simulink model "rSteeringAngle"  (R2024b)
settings: Solver=FixedStepAuto  StartTime=0.0  StopTime=10.0  RelTol=1e-3  EnableMultiTasking=on
undefined symbols (not defined in the file): aSteeringAngleMax, rSteeringAngleGain
settings Model: DataDictionary=Master_Dictionary.sldd  EnableAccessToBaseWorkspace=off  Creator=torni  LastModifiedBy=Will
settings OptimizationCC: DefaultParameterBehavior=Inlined  EnhancedBackFolding=on  PassReuseOutputArgsAs=Individual arguments  ZeroExternalMemoryAtStartup=off  ZeroInternalMemoryAtStartup=off  MaxStackSize=8192  OptimizeBlockOrder=speed  DifferentSizesBufferReuse=on  OptimizationCustomize=off  EfficientTunableParamExpr=on
settings DebuggingCC: ParameterTunabilityLossMsg=error
settings HardwareCC: ProdBitPerPointer=32  ProdBitPerSizeT=32  ProdBitPerPtrDiffT=32  ProdLargestAtomicInteger=Long  ProdLargestAtomicFloat=Double  ProdWordSize=32  ProdLongLongMode=on  ProdHWDeviceType=ARM Compatible->ARM Cortex-M
settings SFSimCC: MATLABDynamicMemAlloc=off
settings RTWCC: Description=Embedded Coder  SystemTargetFile=ert.tlc  HardwareBoard=STM32H7xx Based (Single-core)  TemplateMakefile=ert_default_tmf  Toolchain=GNU Tools for ARM Embedded Processors
settings CodeAppCC: ForceParamTrailComments=on  IgnoreCustomStorageClasses=off  OperatorAnnotations=on  SimulinkDataObjDesc=on  SFDataObjDesc=on  InsertBlockDesc=on
settings ERTTargetCC: TargetLangStandard=C99 (ISO)  CodeReplacementLibrary=ARM Cortex-M  ExtModeTransport=3  ExtModeStaticAlloc=on  ExtModeStaticAllocSize=2048  ExtModeMexFile=ext_xcp  ExtModeIntrfLevel=Level2 - Open

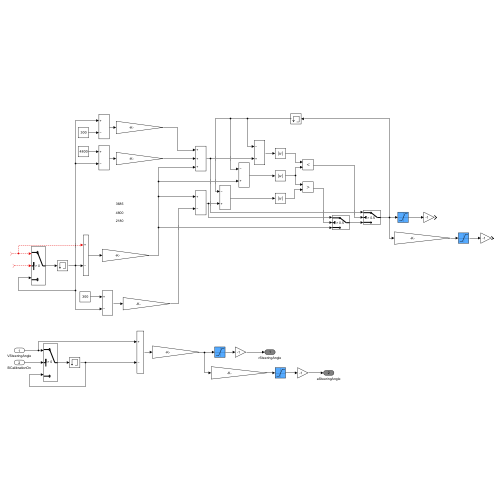
[thumbnail: Simulink's stored preview of the top-level diagram]
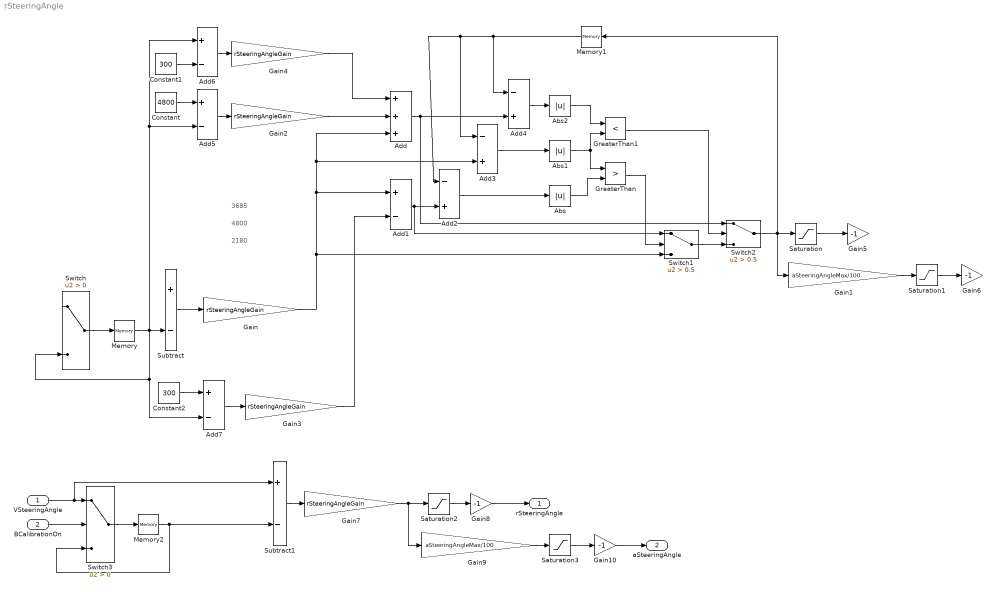
== system rSteeringAngle ==
  note: 4800
  note: 3685
  note: 2180
  VSteeringAngle : Inport  OutDataTypeStr=double
  BCalibrationOn : Inport  Port=2  OutDataTypeStr=boolean
  Abs : Abs  SaturateOnIntegerOverflow=off
  Abs1 : Abs  SaturateOnIntegerOverflow=off
  Abs2 : Abs  SaturateOnIntegerOverflow=off
  Add : Sum  Inputs=+++
  Add{1,5..7} (4 alike) : Sum  Inputs=+-
  Add2 : Sum  Inputs=-+
  Add3 : Sum  Inputs=-+
  Add4 : Sum  Inputs=-+
  Constant : Constant  Value=4800
  Constant1 : Constant  Value=300
  Constant2 : Constant  Value=300
  Gain{,2..4,7} (5 alike) : Gain  Gain=rSteeringAngleGain
  Gain1 : Gain  Gain=aSteeringAngleMax/100
  Gain{5..6,8,10} (4 alike) : Gain  Gain=-1
  Gain9 : Gain  Gain=aSteeringAngleMax/100
  GreaterThan : RelationalOperator  Operator=>  OutDataTypeStr=boolean  RndMeth=Simplest  InputSameDT=off
  GreaterThan1 : RelationalOperator  Operator=<  OutDataTypeStr=boolean  RndMeth=Simplest  InputSameDT=off
  Memory : Memory  InitialCondition=3685  InheritSampleTime=on
  Memory1 : Memory  InheritSampleTime=on
  Memory2 : Memory  InitialCondition=2866  InheritSampleTime=on
  Saturation : Saturate  UpperLimit=100  LowerLimit=-100
  Saturation1 : Saturate  UpperLimit=35  LowerLimit=-35
  Saturation2 : Saturate  UpperLimit=100  LowerLimit=-100
  Saturation3 : Saturate  UpperLimit=35  LowerLimit=-35
  Subtract : Sum  Inputs=+-
  Subtract1 : Sum  Inputs=+-
  Switch : Switch  Criteria=u2 > Threshold  SaturateOnIntegerOverflow=off  InputSameDT=off
  Switch1 : Switch  Criteria=u2 > Threshold  Threshold=0.5  SaturateOnIntegerOverflow=off  InputSameDT=off
  Switch2 : Switch  Criteria=u2 > Threshold  Threshold=0.5  SaturateOnIntegerOverflow=off  InputSameDT=off
  Switch3 : Switch  Criteria=u2 > Threshold  SaturateOnIntegerOverflow=off  InputSameDT=off
  rSteeringAngle : Outport  OutDataTypeStr=double  VectorParamsAs1DForOutWhenUnconnected=off
  aSteeringAngle : Outport  Port=2  OutDataTypeStr=double  VectorParamsAs1DForOutWhenUnconnected=off
  wires:
  ? -> Switch/2
  ? -> Subtract/1, Switch/1
  Switch/1 -> Memory/1
  Memory/1 -> Add6/1, Add5/2, Switch/3, Add7/2, Subtract/2
  Subtract/1 -> Gain/1
  Saturation/1 -> Gain5/1
  Saturation1/1 -> Gain6/1
  Gain1/1 -> Saturation1/1
  Gain/1 -> Add1/1, Add/3, Add3/2, Switch1/3
  Add1/1 -> Switch1/1, Add2/2
  GreaterThan/1 -> Switch1/2
  GreaterThan1/1 -> Switch2/2
  Add/1 -> Add4/2, Switch2/1
  Switch2/1 -> Gain1/1, Memory1/1, Saturation/1
  Memory1/1 -> Add4/1, Add3/1, Add2/1
  Add4/1 -> Abs2/1
  Add3/1 -> Abs1/1
  Add2/1 -> Abs/1
  Abs2/1 -> GreaterThan1/1
  Abs1/1 -> GreaterThan/1, GreaterThan1/2
  Abs/1 -> GreaterThan/2
  Switch1/1 -> Switch2/3
  Constant/1 -> Add5/1
  Add5/1 -> Gain2/1
  Gain2/1 -> Add/2
  Constant1/1 -> Add6/2
  Add6/1 -> Gain4/1
  Gain4/1 -> Add/1
  Add7/1 -> Gain3/1
  Constant2/1 -> Add7/1
  Gain3/1 -> Add1/2
  Subtract1/1 -> Gain7/1
  Memory2/1 -> Subtract1/2, Switch3/3
  Switch3/1 -> Memory2/1
  BCalibrationOn/1 -> Switch3/2
  VSteeringAngle/1 -> Switch3/1, Subtract1/1
  Gain8/1 -> rSteeringAngle/1
  Saturation2/1 -> Gain8/1
  Gain10/1 -> aSteeringAngle/1
  Gain7/1 -> Gain9/1, Saturation2/1
  Gain9/1 -> Saturation3/1
  Saturation3/1 -> Gain10/1
